simulink model "Custom_Analog_Filter"  (R2017a)
settings: Solver=ode15s  StartTime=0.0  StopTime=0.5  MaxStep=0.01  RelTol=1e-3  AbsTol=1e-4  EnableMultiTasking=on
PreLoadFcn:
  | Temperature = 300;
InitFcn:
  | Temperature = str2num(get_param([bdroot '/Temperature'],'Value'));
StopFcn:
  | fg = max(LUT_Resistor_DATA.signals.values(:,2))/max(LUT_Resistor_DATA.signals.values(:,1));
  | disp(['Temperature = ' num2str(Temperature) '; Gain = ' num2str(fg)]);
libraries: fl_lib x13, nesl_utility x3, elec_lib x1
Description:
  | Copyright 2015-2018 The MathWorks, Inc.
settings Model: Creator=smiller  LastModifiedBy=smiller
settings DataIOCC: LimitDataPoints=on  SaveFormat=Array
settings OptimizationCC: ExpressionDepthLimit=2147483647  LifeSpan=inf
settings DebuggingCC: UnderspecifiedInitializationDetection=Classic  MergeDetectMultiDrivingBlocksExec=none  SolverPrmCheckMsg=warning  AllowSymbolicDim=off  StateNameClashWarn=warning  SFUnexpectedBacktrackingDiag=warning  SFNoUnconditionalDefaultTransitionDiag=warning  SFExecutionAtInitializationDiag=none
settings HardwareCC: ProdBitPerPointer=32  ProdBitPerSizeT=32  ProdBitPerPtrDiffT=32  ProdLargestAtomicFloat=None  ProdIntDivRoundTo=Undefined  ProdEndianess=Unspecified  ProdWordSize=32  ProdHWDeviceType=32-bit Generic
settings ModelReferenceCC: PropagateSignalLabelsOutOfModel=off
settings GRTTargetCC: TargetLangStandard=C89/C90 (ANSI)  GeneratePreprocessorConditionals=Disable all
settings ConfigComp: CovMetricSettings=dw  CovHtmlReporting=on  CovSaveCumulativeToWorkspaceVar=on  CovSaveSingleToWorkspaceVar=on  CovExternalEMLEnable=off  CovSFcnEnable=off

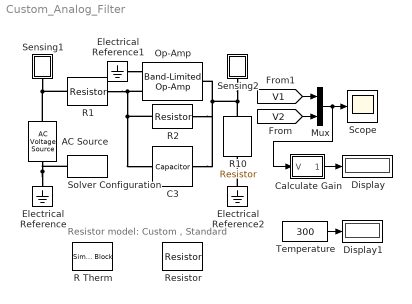
== system Custom_Analog_Filter ==
  note: Resistor model: Custom , Standard
  AC Source : fl_lib/Electrical/Electrical Sources/AC Voltage Source  amp=5 V  shift=0 rad  frequency=60 Hz  omega=20 Hz
  C3 : fl_lib/Electrical/Electrical Elements/Capacitor  c=0.8 uF  r=0.1 Ohm  g=0 1/Ohm  i_specify=off  i_priority=High  i=0 A  i_nominal_specify=off  i_nominal_unit=A  i_nominal_value=1  v_specify=off  v_priority=High  v=0 V  v_nominal_specify=off  v_nominal_unit=V  v_nominal_value=1  vc_specify=on  vc_priority=High  vc=0 V  vc_nominal_specify=off  vc_nominal_unit=V  vc_nominal_value=1
  Calculate Gain : Subsystem
      mask Display: disp('Gain')
  Display : Display
  Display1 : Display
  Electrical Reference : fl_lib/Electrical/Electrical Elements/Electrical Reference
  Electrical Reference1 : fl_lib/Electrical/Electrical Elements/Electrical Reference
  Electrical Reference2 : fl_lib/Electrical/Electrical Elements/Electrical Reference
  Mux : Mux  Inputs=2
  Op-Amp : elec_lib/Integrated Circuits/Band-Limited Op-Amp  A=1000  Rin=1e+06 Ohm  Rout=100 Ohm  Vmin=-5 V  Vmax=5 V  Vdotmax=1000 V/s  f=1e3 Hz  V0=0 V
      settings: SourceProductName=Simscape Electronics  SourceProductBaseCode=SN
  R Therm : SimscapeComponentBlock  SourceFile=MyResistor.MyResistor  ComponentPath=MyResistor.MyResistor  ComponentVariants=MyResistor.MyResistor  ComponentVariantNames=MyResistor  ClassName=MyResistor  SchemaVersion=1  R=10 kOhm  a=0.001 1/K  T0=300 K  T=Temperature K  i_specify=off  i_priority=None  i=0 A  i_nominal_specify=off  i_nominal_unit=A  i_nominal_value=1  v_specify=off  v_priority=None  v=0 V  v_nominal_specify=off  v_nominal_unit=V  v_nominal_value=1
      settings: CopyFcn=simscape.engine.sli.internal.componentblockcallback(gcbh,'COPY')  PreCopyFcn=simscape.engine.sli.internal.componentblockcallback(gcbh,'PRECOPY')  PreDeleteFcn=simscape.engine.sli.internal.componentblockcallback(gcbh,'PREDELETE')
      mask Type: R Therm
  R1 : fl_lib/Electrical/Electrical Elements/Resistor  R=10 kOhm  i_specify=off  i_priority=High  i=0 A  i_nominal_specify=off  i_nominal_unit=A  i_nominal_value=1  v_specify=off  v_priority=High  v=0 V  v_nominal_specify=off  v_nominal_unit=V  v_nominal_value=1
  R10 : fl_lib/Electrical/Electrical Elements/Resistor  R=10 kOhm  i_specify=off  i_priority=High  i=0 A  i_nominal_specify=off  i_nominal_unit=A  i_nominal_value=1  v_specify=off  v_priority=High  v=0 V  v_nominal_specify=off  v_nominal_unit=V  v_nominal_value=1
  R2 : fl_lib/Electrical/Electrical Elements/Resistor  R=10 kOhm  i_specify=off  i_priority=High  i=0 A  i_nominal_specify=off  i_nominal_unit=A  i_nominal_value=1  v_specify=off  v_priority=High  v=0 V  v_nominal_specify=off  v_nominal_unit=V  v_nominal_value=1
  Resistor : fl_lib/Electrical/Electrical Elements/Resistor  R=10 kOhm  i_specify=off  i_priority=High  i=0 A  i_nominal_specify=off  i_nominal_unit=A  i_nominal_value=1  v_specify=off  v_priority=High  v=0 V  v_nominal_specify=off  v_nominal_unit=V  v_nominal_value=1
  Scope : Scope
  Sensing1 : Subsystem
      mask Display: disp('S');
  Sensing2 : Subsystem
      mask Display: disp('S');
  Solver Configuration : nesl_utility/Solver Configuration  PhysicalDomain=network_engine_domain  SubClassName=solver  LeftPortType=input  RightPortType=generic  Accelerate=off  Tones=[]  Harmonics=[]  SimulateNoise=off  Profile=off  UseLocalSampling=off  EnableSwitchedLinearOptims=on  FrequencyDomain=off  UseCCode=off  RelTol=0.001  AbsTol=1e-06  MinStep=1e-09  ToWorkspace=off  RevertToSquareIcSolve=off  NumHomotopyIterations=100  PhasorMode=off  PhasorModeNumHarmonics=1  OverrideAbsTol=off  DoDC=off  ResidualTolerance=1e-9  UseLocalSolver=off  LocalSolverChoice=NE_BACKWARD_EULER_ADVANCER  LocalSolverSampleTime=.001  DoFixedCost=off  MaxNonlinIter=3  MaxModeIter=2  LinearAlgebra=Sparse  DelaysMemoryBudget=1024  AutomaticFiltering=on  FilteringTimeConstant=0.001
  Temperature : Constant  Value=300
  wires:
  Mux/1 -> Calculate Gain/1(V), Scope/1
  [V2] -> Mux/2
  [V1] -> Mux/1
  Calculate Gain/1(Gain) -> Display/1
  Temperature/1 -> Display1/1
  connections:
  R10/LConn1 -- Sensing2/LConn1 -- C3/RConn1 -- R2/RConn1 -- Op-Amp/RConn1
  Op-Amp/LConn2 -- R2/LConn1 -- C3/LConn1 -- R1/RConn1
  Electrical Reference2/LConn1 -- R10/RConn1
  AC Source/RConn1 -- Solver Configuration/RConn1 -- Electrical Reference/LConn1
  AC Source/LConn1 -- R1/LConn1 -- Sensing1/LConn1
  Electrical Reference1/LConn1 -- Op-Amp/LConn1

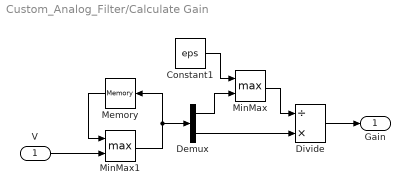
== system Custom_Analog_Filter/Calculate Gain ==
  V : Inport
  Constant1 : Constant  Value=eps
  Demux : Demux  Outputs=2
  Divide : Product  Inputs=/*
  Memory : Memory  X0=[0 0]
  MinMax : MinMax  Function=max  Inputs=2
  MinMax1 : MinMax  Function=max  Inputs=2
  Gain : Outport
  wires:
  MinMax1/1 -> Demux/1, Memory/1
  V/1 -> MinMax1/2
  Demux/2 -> Divide/2
  Divide/1 -> Gain/1
  Demux/1 -> MinMax/2
  MinMax/1 -> Divide/1
  Constant1/1 -> MinMax/1
  Memory/1 -> MinMax1/1

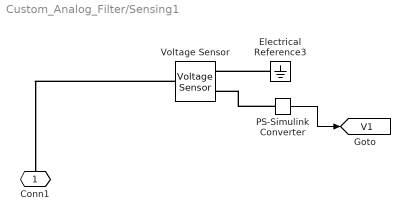
== system Custom_Analog_Filter/Sensing1 ==
  Electrical Reference3 : fl_lib/Electrical/Electrical Elements/Electrical Reference
  PS-Simulink Converter : nesl_utility/PS-Simulink Converter  PhysicalDomain=network_engine_domain  SubClassName=ps_output  LeftPortType=input  RightPortType=output  PseudoPeriodic=off  Frequencies=[]  Unit=1  AffineConversion=off
  Voltage Sensor : fl_lib/Electrical/Electrical Sensors/Voltage Sensor
  Conn1 : PMIOPort  Port=1  Side=Left
  tag scope: V1=global
  wires:
  PS-Simulink Converter/1 -> [V1]
  connections:
  Voltage Sensor/LConn1 -- Conn1/RConn1
  PS-Simulink Converter/LConn1 -- Voltage Sensor/RConn1
  Electrical Reference3/LConn1 -- Voltage Sensor/RConn2

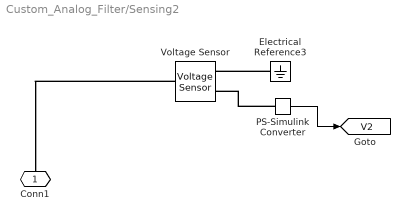
== system Custom_Analog_Filter/Sensing2 ==
  Electrical Reference3 : fl_lib/Electrical/Electrical Elements/Electrical Reference
  PS-Simulink Converter : nesl_utility/PS-Simulink Converter  PhysicalDomain=network_engine_domain  SubClassName=ps_output  LeftPortType=input  RightPortType=output  PseudoPeriodic=off  Frequencies=[]  Unit=1  AffineConversion=off
  Voltage Sensor : fl_lib/Electrical/Electrical Sensors/Voltage Sensor
  Conn1 : PMIOPort  Port=1  Side=Left
  tag scope: V2=global
  wires:
  PS-Simulink Converter/1 -> [V2]
  connections:
  Electrical Reference3/LConn1 -- Voltage Sensor/RConn2
  PS-Simulink Converter/LConn1 -- Voltage Sensor/RConn1
  Voltage Sensor/LConn1 -- Conn1/RConn1
